simulink library "watchdoglib"  (R2015a)
settings: Solver=ode45  StartTime=0.0  StopTime=10.0  RelTol=1e-3
libraries: simulink x2
settings Model: Creator=tkw954  LastModifiedBy=tkw954

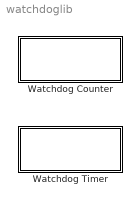
== system watchdoglib ==
  Watchdog Counter : Subsystem  mask(Watchdog){k_max=1e4}
      mask prompts: k_max "Max number of time steps"
      mask help: Halts simulation if the maximum number of time steps is exceeded. Number of steps must be less than 2^32-1.
      mask Help: Travis Wiens t.wiens@usask.ca
      mask Display: fprintf('Max %d steps',k_max)
  Watchdog Timer : Subsystem  mask(Watchdog){dt_max=100}
      mask prompts: dt_max "Max time (s)"
      mask help: Halts simulation if the maximum CPU time is exceeded.
      mask init:
      | t0=cputime;
      mask Help: Travis Wiens t.wiens@usask.ca
      mask Display: fprintf('Max %d s',dt_max)

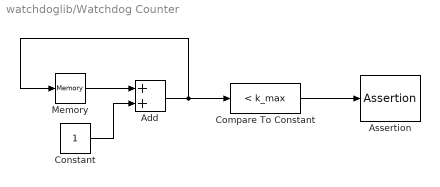
== system watchdoglib/Watchdog Counter ==
  Add : Sum
  Assertion : Assertion
  Compare To Constant : simulink/Logic and Bit Operations/Compare To Constant  relop=<  const=k_max  OutDataTypeStr=boolean
  Constant : Constant
  Memory : Memory  X0=uint32(0)
  wires:
  Constant/1 -> Add/2
  Memory/1 -> Add/1
  Compare To Constant/1 -> Assertion/1
  Add/1 -> Compare To Constant/1, Memory/1

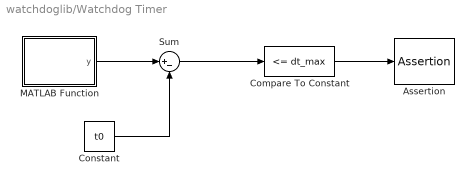
== system watchdoglib/Watchdog Timer ==
  Assertion : Assertion
  Compare To Constant : simulink/Logic and Bit Operations/Compare To Constant  relop=<=  const=dt_max  OutDataTypeStr=boolean
  Constant : Constant  Value=t0
  MATLAB Function : MATLAB Function  TreatAsAtomicUnit=on
  Sum : Sum  Inputs=|+-
  wires:
  Sum/1 -> Compare To Constant/1
  Constant/1 -> Sum/2
  MATLAB Function/1(y) -> Sum/1
  Compare To Constant/1 -> Assertion/1

== matlab function watchdoglib/Watchdog Timer/MATLAB Function ==
  data: y output
function y = fcn()
%#codegen
coder.extrinsic('cputime')
 y=nan;
y = cputime;
